simulink model "upconverst"  (R2021a)
settings: Solver=VariableStepAuto  StartTime=0.0  StopTime=1000.0  RelTol=1e-3
libraries: dsp_blocks x5
settings Model: Creator=nathanalemayehu  LastModifiedBy=nathanalemayehu

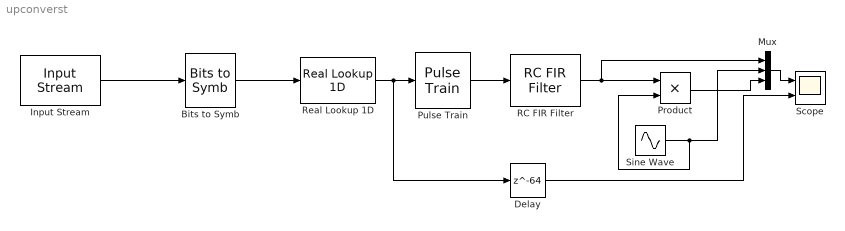
== system upconverst ==
  Bits to Symb : dsp_blocks/Conversions/Bits to Symb
  Delay : Delay  DelayLength=64
  Input Stream : dsp_blocks/Sources//Sinks/Input Stream  period=10  width=1  fname=rand.mat
  Mux : Mux  Inputs=3
  Product : Product
  Pulse Train : dsp_blocks/Conversions/Pulse Train  period=10
  RC FIR Filter : dsp_blocks/Filters/RC FIR Filter  period=10  beta=0.5  root=off  filt_len=128  win_type=on
  Real Lookup 1D : dsp_blocks/Conversions/Real Lookup 1D  table=[-1 1]
  Scope : Scope  NumInputPorts=2
  Sine Wave : Sin  SampleTime=0
  wires:
  Input Stream/1 -> Bits to Symb/1
  Real Lookup 1D/1 -> Delay/1, Pulse Train/1
  Pulse Train/1 -> RC FIR Filter/1
  Bits to Symb/1 -> Real Lookup 1D/1
  Delay/1 -> Scope/2
  RC FIR Filter/1 -> Mux/1, Product/1
  Mux/1 -> Scope/1
  Sine Wave/1 -> Mux/2, Product/2
  Product/1 -> Mux/3
